simulink model "bldc_three_loop_PI"  (R2022a)
settings: Solver=ode45  StartTime=0.0  StopTime=4  RelTol=1e-3  EnableMultiTasking=on
undefined symbols (not defined in the file): sigbuilder_block
libraries: simulink x9, spsPermanentMagnetSynchronousMachineLib x1, spsDCVoltageSourceLib x1, spsUniversalBridgeLib x1, spspowerguiLib x1
settings Model: Creator=Administrator  LastModifiedBy=28061
settings SolverCC: MaxConsecutiveMinStep=10  ZeroCrossAlgorithm=Adaptive  AlgebraicLoopSolver=TrustRegion
settings DataIOCC: LimitDataPoints=on  SaveFormat=Array  SignalLoggingSaveFormat=ModelDataLogs  ReturnWorkspaceOutputs=off
settings OptimizationCC: ExpressionDepthLimit=2147483647  LifeSpan=inf
settings DebuggingCC: AlgebraicLoopMsg=none  UnderspecifiedInitializationDetection=Classic  MergeDetectMultiDrivingBlocksExec=none  FcnCallInpInsideContextMsg=warning  AllowSymbolicDim=off  StateNameClashWarn=warning  SFUnexpectedBacktrackingDiag=warning  SFNoUnconditionalDefaultTransitionDiag=warning  SFExecutionAtInitializationDiag=none  SFMachineParentedDataDiag=warning  ArithmeticOperatorsInVariantConditions=warning
settings HardwareCC: ProdBitPerPointer=32  ProdBitPerSizeT=32  ProdBitPerPtrDiffT=32  ProdLargestAtomicFloat=None  ProdIntDivRoundTo=Undefined  ProdEndianess=Unspecified  ProdWordSize=32  ProdHWDeviceType=32-bit Generic
settings ModelReferenceCC: PropagateSignalLabelsOutOfModel=off
settings SFSimCC: SimUseLocalCustomCode=off  CustomCodeUndefinedFunction=UseInterfaceOnly
settings RTWCC: RTWUseLocalCustomCode=off
settings CodeAppCC: StateflowObjectComments=on
settings GRTTargetCC: TargetLangStandard=C89/C90 (ANSI)  CombineOutputUpdateFcns=off  GRTInterface=on
settings ConfigComp: CovMetricSettings=dw  CovSaveCumulativeToWorkspaceVar=on  CovSaveSingleToWorkspaceVar=on  CovExternalEMLEnable=off
settings SimscapeCC: SimscapeNormalizeSystem=off

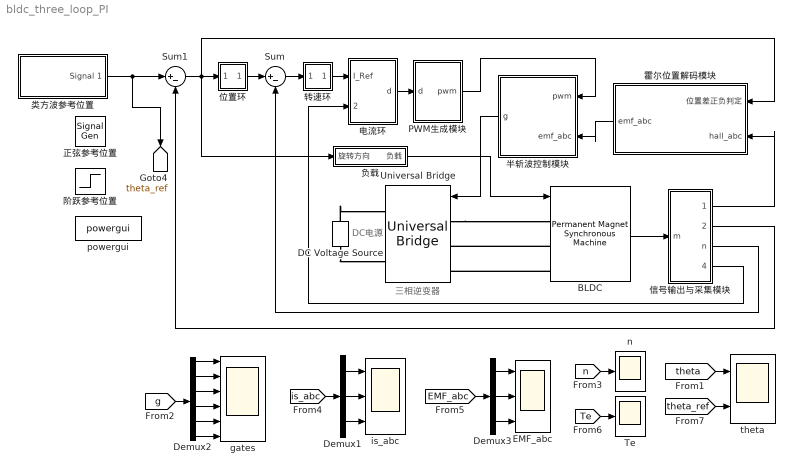
== system bldc_three_loop_PI ==
  note: DC电源
  note: 三相逆变器
  BLDC : spsPermanentMagnetSynchronousMachineLib/Permanent Magnet Synchronous Machine  NbPhases=3  FluxDistribution=Trapezoidal  RotorType=Round  MechanicalLoad=Torque Tm  PresetModel=No  ShowDetailedParameters=on  MeasurementBus=off  Resistance=1.03  Inductance=820e-6  dqInductances=[8.5e-3,8.5e-3]  La=0.000395  MachineConstant=Voltage Constant (V_peak L-L / krpm)  Flux=0.073456  VoltageCst=15.3846  TorqueCst=0.14691  Flat=120  Mechanical=[0.0000831 0.0001 1 0]  PolePairs=4  InitialConditions=[0,0, 0,0]  InitialConditions5ph=[0 0 0 0 0 0]  RefAngle=Aligned with phase A axis (original Park)  IterativeDiscreteModel=Trapezoidal non iterative  TsBlock=-1  TsPowergui=0
  DC Voltage Source : spsDCVoltageSourceLib/DC Voltage Source  Amplitude=48  Measurements=None
  Demux1 : Demux  Outputs=3
  Demux2 : Demux  Outputs=6
  Demux3 : Demux  Outputs=3
  EMF_abc : Scope  NumInputPorts=3
  PWM生成模块 : Subsystem
  Sum : Sum  Inputs=|+-
  Sum1 : Sum  Inputs=|+-
  Te : Scope
  Universal Bridge : spsUniversalBridgeLib/Universal Bridge  Arms=3  SnubberResistance=1e5  SnubberCapacitance=inf  Device=MOSFET / Diodes  Ron=1e-3  Lon=0  ForwardVoltages="[  0  0  ]"  ForwardVoltage=0  GTOparameters=[ 10e-6 , 20e-6 ]  IGBTparameters=[ 1e-6 , 2e-6 ]  Measurements=None  Measurements_2=None  converterType=Rectifier
  gates : Scope  NumInputPorts=6
  is_abc : Scope  NumInputPorts=3
  n : Scope
  powergui : spspowerguiLib/powergui  Priority=1  SimulationMode=Discrete  SampleTime=5e-5  frequency=60  Iterations=50  frequencyindice=0  Pbase=100e6  ErrMax=1e-4  UnitsV=kV  UnitsW=MW  buscounter=0  FunctionMessages=off  echomessages=off  EnableUseOfTLC=off  CurrentSourceSwitches=off  DisableSnubberDevices=off  DisableRonSwitches=off  DisableVfSwitches=off  DisplayEquations=off  AutomaticDiscreteSolvers=off  SolverType=Tustin/Backward Euler (TBE)  Interpol=off  ExternalGateDelay=off  methode=off  Ts=10  x0status=blocks  SPID=off  SwTol=0  HookPort=off  NonlinearTolerance=1e-4  nMaxIteration=100  ContinueOnMaxIteration=off  RestoreLinks=warning  ResistiveCurrentMeasurement=off  Frange=[0:2:500]  Ylog=off  Xlog=on  ShowGrid=off  save=off  variable=ZData  structure=0  ZoomFFT=off  StartTime=0.0  cycles=1  DisplayStyle=1  fundamental=60  FreqAxis=off  MaxFrequency=1000  frequencyindicesteady=1  RmsSteady=1  display=off
  theta : Scope  NumInputPorts=2
  位置环 : Subsystem
      mask Display: fprintf('PI')
  信号输出与采集模块 : Subsystem
  半斩波控制模块 : Subsystem
  正弦参考位置 : SignalGenerator  Amplitude=30  Frequency=0.2
  "电流环 " : Subsystem
      mask Display: fprintf('PI')
  类方波参考位置 : Subsystem  Tag=STV Subsys  LoadFcn=sigbuilder_block('load');  StartFcn=sigbuilder_block('start');  StopFcn=sigbuilder_block('stop');  ClipboardFcn=sigbuilder_block('clipboard');  mask(Sigbuilder block){tuvar=[0:10]}
      mask help: Simulink:masks:SigbuilderBlock_MD
      mask init:
      | if ~strcmp(get_param(bdroot(gcbh),'SimulationStatus'),'stopped') tuvar = sigbuilder_block('maskInit'); end
      settings: CopyFcn=sigbuilder_block('copy');  DeleteFcn=sigbuilder_block('delete');  ModelCloseFcn=sigbuilder_block('modelClose');  PreSaveFcn=sigbuilder_block('preSave');  PauseFcn=sigbuilder_block('pause');  ContinueFcn=sigbuilder_block('continue');  NameChangeFcn=sigbuilder_block('namechange');  OpenFcn=sigbuilder_block('open',[426 176 550.5 326 ]);  CloseFcn=sigbuilder_block('close');
      mask Display: plot(0, 0, 100, 100,[2, 2, 32, 32, 2], [68, 8, 8, 68, 68],[32, 2], [38, 38], [32, 19, 2],[53, 60, 44], [32, 17, 17, 2],[16, 16, 31, 31]);txt = getActiveGroup(gcbh);text(2, 100, txt,'verticalAlignment', 'top');
  负载 : Subsystem
  转速环 : Subsystem
      mask Display: fprintf('PI')
  阶跃参考位置 : Step  Time=0.3  After=-30  SampleTime=0
  霍尔位置解码模块 : Subsystem
  tag scope: theta_ref=global
  wires:
  转速环/1(i_Ref) -> "电流环 "/1(I_Ref)
  BLDC/1 -> 信号输出与采集模块/1(m)
  信号输出与采集模块/4(is_abc) -> "电流环 "/2(is_abc)
  Demux2/2 -> gates/2
  Demux2/3 -> gates/3
  Demux2/5 -> gates/5
  Demux2/4 -> gates/4
  Demux2/1 -> gates/1
  Demux2/6 -> gates/6
  [g] -> Demux2/1
  [n] -> n/1
  Demux1/2 -> is_abc/2
  Demux1/1 -> is_abc/1
  Demux1/3 -> is_abc/3
  [is_abc] -> Demux1/1
  [EMF_abc] -> Demux3/1
  Demux3/3 -> EMF_abc/3
  Demux3/1 -> EMF_abc/1
  Demux3/2 -> EMF_abc/2
  [Te] -> Te/1
  信号输出与采集模块/3(n) -> Sum/2
  "电流环 "/1(d) -> PWM生成模块/1(d)
  半斩波控制模块/1(g) -> Universal Bridge/1
  PWM生成模块/1(pwm) -> 半斩波控制模块/1(pwm)
  Sum1/1 -> 霍尔位置解码模块/1(位置差正负判定), 负载/1(旋转方向), 位置环/1(err)
  信号输出与采集模块/2(theta) -> Sum1/2
  类方波参考位置/1(Signal 1) -> [theta_ref], Sum1/1
  [theta] -> theta/1
  [theta_ref] -> theta/2
  位置环/1(i_Ref) -> Sum/1
  Sum/1 -> 转速环/1(err)
  信号输出与采集模块/1(hall_abc) -> 霍尔位置解码模块/2(hall_abc)
  霍尔位置解码模块/1(emf_abc) -> 半斩波控制模块/2("emf_abc ")
  负载/1(负载) -> BLDC/1
  connections:
  DC Voltage Source/RConn1 -- Universal Bridge/RConn1
  DC Voltage Source/LConn1 -- Universal Bridge/RConn2
  Universal Bridge/LConn1 -- BLDC/LConn1
  BLDC/LConn2 -- Universal Bridge/LConn2
  BLDC/LConn3 -- Universal Bridge/LConn3

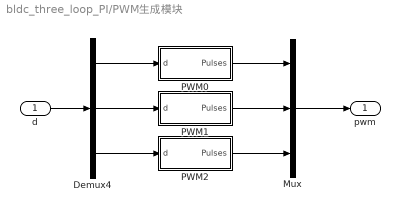
== system bldc_three_loop_PI/PWM生成模块 ==
  d : Inport
  Demux4 : Demux  Outputs=3
  Mux : Mux  Inputs=3
  PWM0 : Subsystem
  PWM1 : Subsystem
  PWM2 : Subsystem
  pwm : Outport  VectorParamsAs1DForOutWhenUnconnected=off
  wires:
  Demux4/1 -> PWM0/1("d ")
  PWM0/1(Pulses) -> Mux/1
  Demux4/2 -> PWM1/1("d ")
  PWM1/1(Pulses) -> Mux/2
  Demux4/3 -> PWM2/1("d ")
  PWM2/1(Pulses) -> Mux/3
  d/1 -> Demux4/1
  Mux/1 -> pwm/1

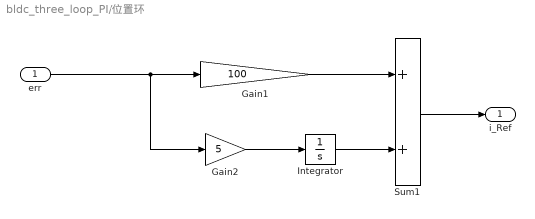
== system bldc_three_loop_PI/位置环 ==
  err : Inport
  Gain1 : Gain  Gain=100
  Gain2 : Gain  Gain=5
  Integrator : Integrator
  Sum1 : Sum
  i_Ref : Outport  VectorParamsAs1DForOutWhenUnconnected=off
  wires:
  err/1 -> Gain1/1, Gain2/1
  Sum1/1 -> i_Ref/1
  Integrator/1 -> Sum1/2
  Gain2/1 -> Integrator/1
  Gain1/1 -> Sum1/1

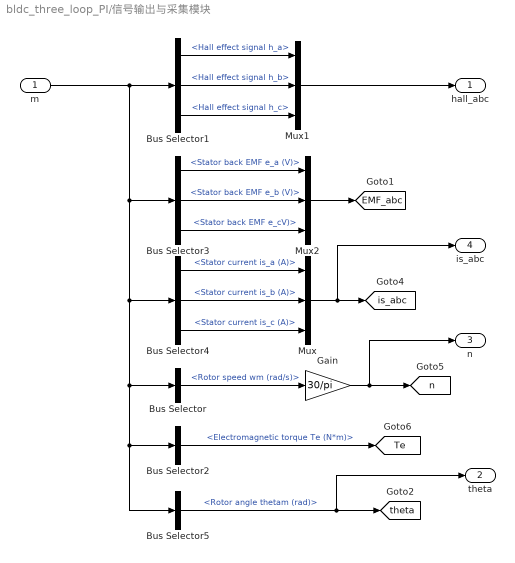
== system bldc_three_loop_PI/信号输出与采集模块 ==
  m : Inport
  Bus Selector : BusSelector  OutputSignals=Rotor speed wm (rad/s)
  Bus Selector1 : BusSelector  OutputSignals=Hall effect signal h_a,Hall effect signal h_b,Hall effect signal h_c
  Bus Selector2 : BusSelector  OutputSignals=Electromagnetic torque Te (N*m)
  Bus Selector3 : BusSelector  OutputSignals=Stator back EMF e_a (V),Stator back EMF e_b (V),Stator back EMF e_cV)
  Bus Selector4 : BusSelector  OutputSignals=Stator current is_a (A),Stator current is_b (A),Stator current is_c (A)
  Bus Selector5 : BusSelector  OutputSignals=Rotor angle thetam (rad)
  Gain : Gain  Gain=30/pi
  Mux : Mux  Inputs=3
  Mux1 : Mux  Inputs=3
  Mux2 : Mux  Inputs=3
  hall_abc : Outport  VectorParamsAs1DForOutWhenUnconnected=off
  theta : Outport  Port=2  VectorParamsAs1DForOutWhenUnconnected=off
  n : Outport  Port=3  VectorParamsAs1DForOutWhenUnconnected=off
  is_abc : Outport  Port=4  VectorParamsAs1DForOutWhenUnconnected=off
  tag scope: EMF_abc=global, Te=global, is_abc=global, n=global, theta=global
  wires:
  Bus Selector/1 -> Gain/1  "<Rotor speed wm (rad/s)>"
  Gain/1 -> [n], n/1
  Bus Selector3/1 -> Mux2/1  "<Stator back EMF e_a (V)>"
  Bus Selector3/2 -> Mux2/2  "<Stator back EMF e_b (V)>"
  Bus Selector3/3 -> Mux2/3  "<Stator back EMF e_cV)>"
  Bus Selector4/1 -> Mux/1  "<Stator current is_a (A)>"
  Bus Selector4/2 -> Mux/2  "<Stator current is_b (A)>"
  Bus Selector4/3 -> Mux/3  "<Stator current is_c (A)>"
  Mux/1 -> [is_abc], is_abc/1
  Bus Selector2/1 -> [Te]  "<Electromagnetic torque Te (N*m)>"
  Bus Selector1/2 -> Mux1/2  "<Hall effect signal h_b>"
  Bus Selector1/1 -> Mux1/1  "<Hall effect signal h_a>"
  Bus Selector1/3 -> Mux1/3  "<Hall effect signal h_c>"
  Mux1/1 -> hall_abc/1
  Mux2/1 -> [EMF_abc]
  m/1 -> Bus Selector4/1, Bus Selector5/1, Bus Selector2/1, Bus Selector/1, Bus Selector3/1, Bus Selector1/1
  Bus Selector5/1 -> theta/1, [theta]  "<Rotor angle thetam (rad)>"

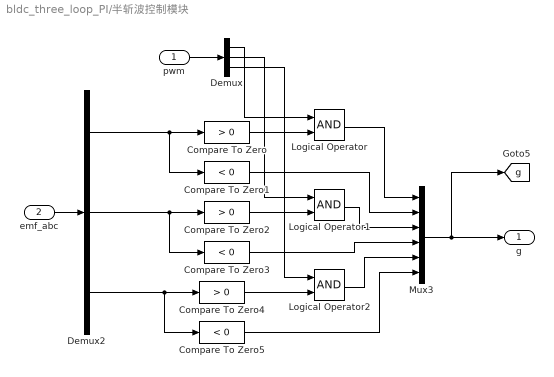
== system bldc_three_loop_PI/半斩波控制模块 ==
  pwm : Inport
  "emf_abc " : Inport  Port=2
  Compare To Zero : simulink/Logic and Bit Operations/Compare To Zero  relop=>  OutDataTypeStr=boolean  ZeroCross=off
  Compare To Zero1 : simulink/Logic and Bit Operations/Compare To Zero  relop=<  OutDataTypeStr=boolean  ZeroCross=off
  Compare To Zero2 : simulink/Logic and Bit Operations/Compare To Zero  relop=>  OutDataTypeStr=boolean  ZeroCross=off
  Compare To Zero3 : simulink/Logic and Bit Operations/Compare To Zero  relop=<  OutDataTypeStr=boolean  ZeroCross=off
  Compare To Zero4 : simulink/Logic and Bit Operations/Compare To Zero  relop=>  OutDataTypeStr=boolean  ZeroCross=off
  Compare To Zero5 : simulink/Logic and Bit Operations/Compare To Zero  relop=<  OutDataTypeStr=boolean  ZeroCross=off
  Demux : Demux  Outputs=3
  Demux2 : Demux  Outputs=3
  Logical Operator : Logic  AllPortsSameDT=off  OutDataTypeStr=boolean
  Logical Operator1 : Logic  AllPortsSameDT=off  OutDataTypeStr=boolean
  Logical Operator2 : Logic  AllPortsSameDT=off  OutDataTypeStr=boolean
  Mux3 : Mux  Inputs=6
  g : Outport  VectorParamsAs1DForOutWhenUnconnected=off
  tag scope: g=global
  wires:
  Compare To Zero5/1 -> Mux3/6
  Compare To Zero3/1 -> Mux3/4
  Demux2/3 -> Compare To Zero5/1, Compare To Zero4/1
  Demux2/2 -> Compare To Zero3/1, Compare To Zero2/1
  Demux2/1 -> Compare To Zero1/1, Compare To Zero/1
  "emf_abc "/1 -> Demux2/1
  Compare To Zero/1 -> Logical Operator/2
  Compare To Zero1/1 -> Mux3/2
  Logical Operator/1 -> Mux3/1
  Compare To Zero2/1 -> Logical Operator1/2
  Compare To Zero4/1 -> Logical Operator2/2
  Logical Operator1/1 -> Mux3/3
  Logical Operator2/1 -> Mux3/5
  pwm/1 -> Demux/1
  Demux/1 -> Logical Operator/1
  Demux/2 -> Logical Operator1/1
  Demux/3 -> Logical Operator2/1
  Mux3/1 -> [g], g/1

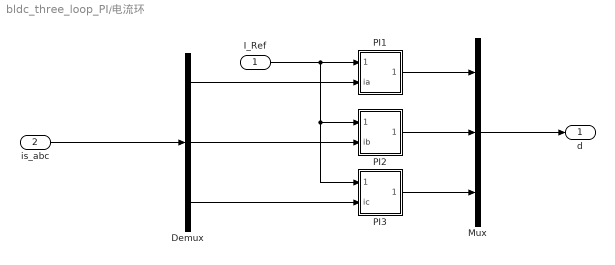
== system bldc_three_loop_PI/电流环  ==
  I_Ref : Inport
  is_abc : Inport  Port=2
  Demux : Demux  Outputs=3
  Mux : Mux  Inputs=3
  PI1 : Subsystem
  PI2 : Subsystem
  PI3 : Subsystem
  d : Outport  VectorParamsAs1DForOutWhenUnconnected=off
  wires:
  PI1/1(Out1) -> Mux/1
  PI2/1(Out1) -> Mux/2
  PI3/1(Out1) -> Mux/3
  I_Ref/1 -> PI3/1(iRef), PI2/1(iRef), PI1/1(iRef)
  Mux/1 -> d/1
  Demux/1 -> PI1/2(ia)
  Demux/2 -> PI2/2(ib)
  Demux/3 -> PI3/2(ic)
  is_abc/1 -> Demux/1

== system bldc_three_loop_PI/类方波参考位置 ==
  Demux : Demux  Tag=STV Demux  Outputs=1
      settings: DisplayOption=none
  FromWs : FromWorkspace  Tag=STV FromWs  VariableName=tuvar
      SigBuilderData=|
      | common.afterFinalStr = 'Extrapolate'
      | common.sampleTime = 0
      | dataSet.timeRange = [0 10]
      | dataSet.name = 'Group 1'
      | sbobj.Groups.Name = 'Group 1'
      | sbobj.Groups.Signals.Name = 'Signal 1'
      | sbobj.Groups.Signals.XData = [0 0.5 0.5 1 1 1.5 1.5 2 2 3 3 3.5 3.5 10]
      | sbobj.Groups.Signals.YData = [0 0 30 30 0 0 -30 -30 40 40 15 15 0 0]
  Signal 1 : Outport  Tag=STV Outport
  wires:
  Demux/1 -> Signal 1/1
  FromWs/1 -> Demux/1

== system bldc_three_loop_PI/负载 ==
  旋转方向 : Inport
  Constant : Constant  Value=-0.25
  Constant1 : Constant  Value=0.25
  正反转切换 : Switch  Criteria=u2 > Threshold  SaturateOnIntegerOverflow=off  InputSameDT=off
  负载 : Outport
  wires:
  Constant1/1 -> 正反转切换/3
  Constant/1 -> 正反转切换/1
  旋转方向/1 -> 正反转切换/2
  正反转切换/1 -> 负载/1

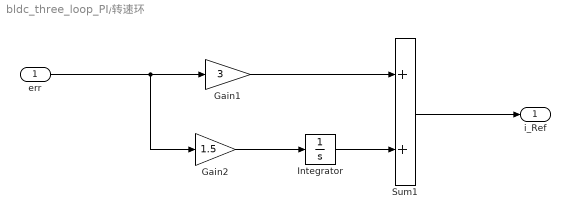
== system bldc_three_loop_PI/转速环 ==
  err : Inport
  Gain1 : Gain  Gain=3
  Gain2 : Gain  Gain=1.5
  Integrator : Integrator
  Sum1 : Sum
  i_Ref : Outport  VectorParamsAs1DForOutWhenUnconnected=off
  wires:
  Gain1/1 -> Sum1/1
  Gain2/1 -> Integrator/1
  Integrator/1 -> Sum1/2
  Sum1/1 -> i_Ref/1
  err/1 -> Gain2/1, Gain1/1

== system bldc_three_loop_PI/霍尔位置解码模块 ==
  位置差正负判定 : Inport
  hall_abc : Inport  Port=2
  反转逻辑 : Subsystem
  正反转切换 : Switch  Criteria=u2 > Threshold  SaturateOnIntegerOverflow=off  InputSameDT=off
  正转逻辑 : Subsystem
  emf_abc : Outport
  wires:
  正转逻辑/1(emf_abc) -> 正反转切换/1  "emf_abc"
  反转逻辑/1(emf_abc) -> 正反转切换/3  "emf_abc"
  hall_abc/1 -> 反转逻辑/1(hall_abc), 正转逻辑/1(hall_abc)
  正反转切换/1 -> emf_abc/1
  位置差正负判定/1 -> 正反转切换/2

== system bldc_three_loop_PI/PWM生成模块/PWM0 ==
  "d " : Inport
  Data Type Conversion1 : DataTypeConversion  OutDataTypeStr=boolean
  Data Type Conversion : DataTypeConversion  SaturateOnIntegerOverflow=off  RndMeth=Floor
  Relational Operator : RelationalOperator  ZeroCross=off
  Triangle : simulink/Sources/Repeating Sequence  rep_seq_t=[0 1/30000/4 2/30000/4 3/30000/4 1/30000]  rep_seq_y=[0 1 0 -1 0]
  Pulses : Outport  VectorParamsAs1DForOutWhenUnconnected=off
  wires:
  Triangle/1 -> Relational Operator/2
  "d "/1 -> Relational Operator/1
  Relational Operator/1 -> Data Type Conversion/1
  Data Type Conversion/1 -> Data Type Conversion1/1
  Data Type Conversion1/1 -> Pulses/1

== system bldc_three_loop_PI/PWM生成模块/PWM1 ==
  "d " : Inport
  Data Type Conversion1 : DataTypeConversion  OutDataTypeStr=boolean
  Data Type Conversion : DataTypeConversion  SaturateOnIntegerOverflow=off  RndMeth=Floor
  Relational Operator : RelationalOperator  ZeroCross=off
  Triangle : simulink/Sources/Repeating Sequence  rep_seq_t=[0 1/30000/4 2/30000/4 3/30000/4 1/30000]  rep_seq_y=[0 1 0 -1 0]
  Pulses : Outport  VectorParamsAs1DForOutWhenUnconnected=off
  wires:
  Data Type Conversion1/1 -> Pulses/1
  Data Type Conversion/1 -> Data Type Conversion1/1
  Relational Operator/1 -> Data Type Conversion/1
  "d "/1 -> Relational Operator/1
  Triangle/1 -> Relational Operator/2

== system bldc_three_loop_PI/PWM生成模块/PWM2 ==
  "d " : Inport
  Data Type Conversion1 : DataTypeConversion  OutDataTypeStr=boolean
  Data Type Conversion : DataTypeConversion  SaturateOnIntegerOverflow=off  RndMeth=Floor
  Relational Operator : RelationalOperator  ZeroCross=off
  Triangle : simulink/Sources/Repeating Sequence  rep_seq_t=[0 1/30000/4 2/30000/4 3/30000/4 1/30000]  rep_seq_y=[0 1 0 -1 0]
  Pulses : Outport  VectorParamsAs1DForOutWhenUnconnected=off
  wires:
  Triangle/1 -> Relational Operator/2
  "d "/1 -> Relational Operator/1
  Relational Operator/1 -> Data Type Conversion/1
  Data Type Conversion/1 -> Data Type Conversion1/1
  Data Type Conversion1/1 -> Pulses/1

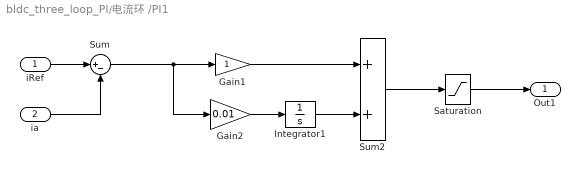
== system bldc_three_loop_PI/电流环 /PI1 ==
  iRef : Inport
  ia : Inport  Port=2
  Gain1 : Gain
  Gain2 : Gain  Gain=0.01
  Integrator1 : Integrator
  Saturation : Saturate  UpperLimit=1  LowerLimit=-1  ZeroCross=off
  Sum : Sum  Inputs=|+-
  Sum2 : Sum
  Out1 : Outport  VectorParamsAs1DForOutWhenUnconnected=off
  wires:
  Saturation/1 -> Out1/1
  ia/1 -> Sum/2
  iRef/1 -> Sum/1
  Sum2/1 -> Saturation/1
  Integrator1/1 -> Sum2/2
  Gain2/1 -> Integrator1/1
  Gain1/1 -> Sum2/1
  Sum/1 -> Gain1/1, Gain2/1

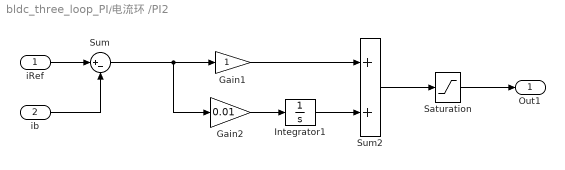
== system bldc_three_loop_PI/电流环 /PI2 ==
  iRef : Inport
  ib : Inport  Port=2
  Gain1 : Gain
  Gain2 : Gain  Gain=0.01
  Integrator1 : Integrator
  Saturation : Saturate  UpperLimit=1  LowerLimit=-1  ZeroCross=off
  Sum : Sum  Inputs=|+-
  Sum2 : Sum
  Out1 : Outport  VectorParamsAs1DForOutWhenUnconnected=off
  wires:
  iRef/1 -> Sum/1
  ib/1 -> Sum/2
  Saturation/1 -> Out1/1
  Sum/1 -> Gain1/1, Gain2/1
  Sum2/1 -> Saturation/1
  Gain1/1 -> Sum2/1
  Gain2/1 -> Integrator1/1
  Integrator1/1 -> Sum2/2

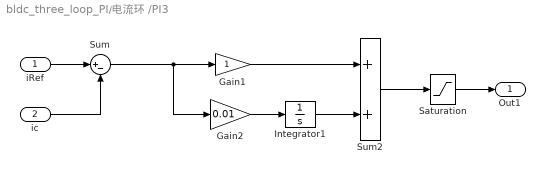
== system bldc_three_loop_PI/电流环 /PI3 ==
  iRef : Inport
  ic : Inport  Port=2
  Gain1 : Gain
  Gain2 : Gain  Gain=0.01
  Integrator1 : Integrator
  Saturation : Saturate  UpperLimit=1  LowerLimit=-1  ZeroCross=off
  Sum : Sum  Inputs=|+-
  Sum2 : Sum
  Out1 : Outport  VectorParamsAs1DForOutWhenUnconnected=off
  wires:
  Saturation/1 -> Out1/1
  ic/1 -> Sum/2
  iRef/1 -> Sum/1
  Sum/1 -> Gain1/1, Gain2/1
  Sum2/1 -> Saturation/1
  Gain1/1 -> Sum2/1
  Gain2/1 -> Integrator1/1
  Integrator1/1 -> Sum2/2

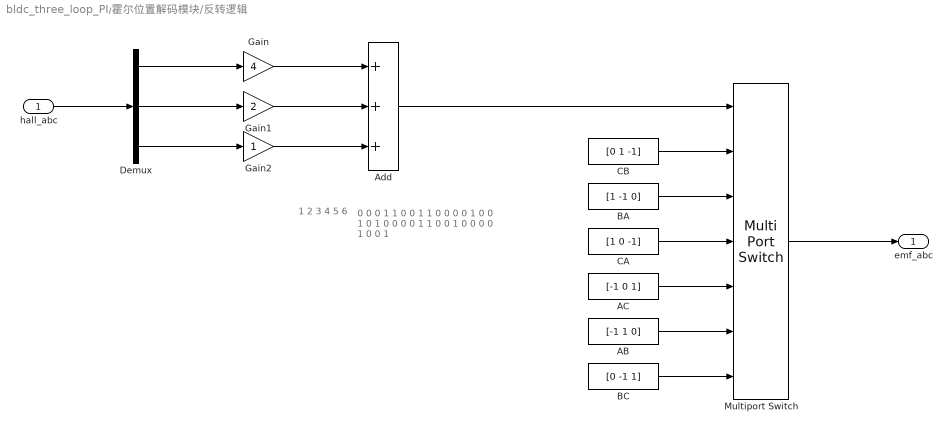
== system bldc_three_loop_PI/霍尔位置解码模块/反转逻辑 ==
  note: 0 0 0 1 1 0
      | 0 1 1 0 0 0
      | 0 1 0 0 1 0
      | 1 0 0 0 0 1
      | 1 0 0 1 0 0
      | 0 0 1 0 0 1
  note: 1
      | 2
      | 3
      | 4
      | 5
      | 6
  hall_abc : Inport
  AB : Constant  Value=[-1 1 0]
  AC : Constant  Value=[-1 0 1]
  Add : Sum  Inputs=+++
  BA : Constant  Value=[1 -1 0]
  BC : Constant  Value=[0 -1 1]
  CA : Constant  Value=[1 0 -1]
  CB : Constant  Value=[0 1 -1]
  Demux : Demux  Outputs=3
  Gain : Gain  Gain=4
  Gain1 : Gain  Gain=2
  Gain2 : Gain
  Multiport Switch : MultiPortSwitch  Inputs=6  SaturateOnIntegerOverflow=off  InputSameDT=off
  emf_abc : Outport
  wires:
  BA/1 -> Multiport Switch/3
  CB/1 -> Multiport Switch/2
  CA/1 -> Multiport Switch/4
  AB/1 -> Multiport Switch/6
  BC/1 -> Multiport Switch/7
  Multiport Switch/1 -> emf_abc/1
  Add/1 -> Multiport Switch/1
  AC/1 -> Multiport Switch/5
  Gain/1 -> Add/1
  Gain1/1 -> Add/2
  Gain2/1 -> Add/3
  Demux/2 -> Gain1/1
  Demux/1 -> Gain/1
  Demux/3 -> Gain2/1
  hall_abc/1 -> Demux/1

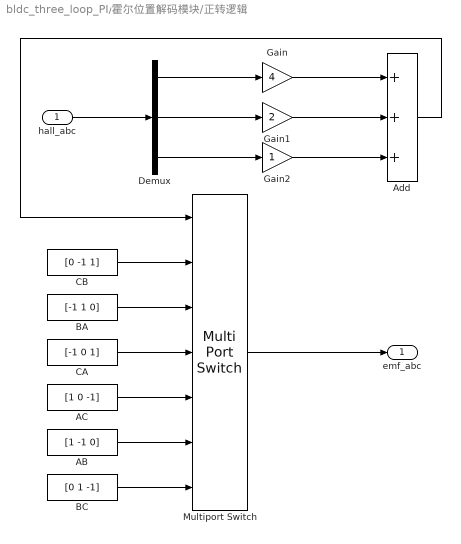
== system bldc_three_loop_PI/霍尔位置解码模块/正转逻辑 ==
  hall_abc : Inport
  AB : Constant  Value=[1 -1 0]
  AC : Constant  Value=[1 0 -1]
  Add : Sum  Inputs=+++
  BA : Constant  Value=[-1 1 0]
  BC : Constant  Value=[0 1 -1]
  CA : Constant  Value=[-1 0 1]
  CB : Constant  Value=[0 -1 1]
  Demux : Demux  Outputs=3
  Gain : Gain  Gain=4
  Gain1 : Gain  Gain=2
  Gain2 : Gain
  Multiport Switch : MultiPortSwitch  Inputs=6  SaturateOnIntegerOverflow=off  InputSameDT=off
  emf_abc : Outport
  wires:
  BA/1 -> Multiport Switch/3
  CB/1 -> Multiport Switch/2
  CA/1 -> Multiport Switch/4
  AB/1 -> Multiport Switch/6
  BC/1 -> Multiport Switch/7
  Multiport Switch/1 -> emf_abc/1
  Add/1 -> Multiport Switch/1
  AC/1 -> Multiport Switch/5
  Gain/1 -> Add/1
  Gain1/1 -> Add/2
  Gain2/1 -> Add/3
  Demux/2 -> Gain1/1
  Demux/1 -> Gain/1
  Demux/3 -> Gain2/1
  hall_abc/1 -> Demux/1
